simulink model "simulation"  (R2023a)
settings: Solver=ode4  StartTime=0.0  StopTime=simulation_time_end  FixedStep=simulation_time_step  RelTol=1e-3
values from neighbouring files (symbols this model uses):
  b = 0.0043    [code_Q2.m]
  J = 0.005    [code_Q2.m]
  K_b = 0.024    [code_Q2.m]
  K_m = 24e-3    (= 0.024)    [code_Q2.m]
  K_p = my_K_p    [code_Q2.m]
  K_u = 1.2    [code_Q2.m]
  L_a = 0.26e-3    (= 0.00026)    [code_Q2.m]
  N_r = 4.9    [code_Q2.m]
  R_a = 2.2    [code_Q2.m]
  simulation_time_start = 1    [code_Q2.m]
  T_d = 0    [code_Q2.m]
  theta_ref = pi/4    (= 0.785398163397)    [code_Q2.m]
settings Model: Creator=אלמוג  LastModifiedBy=אלמוג

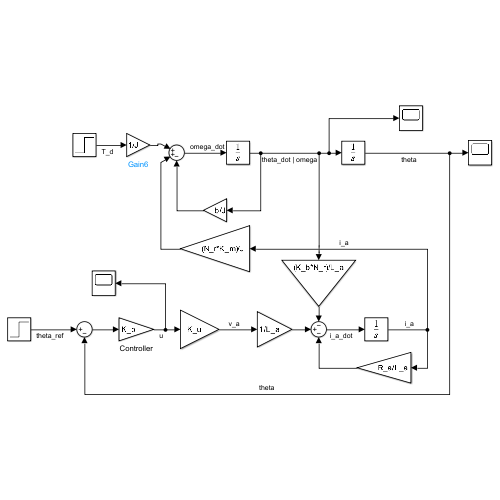
[thumbnail: Simulink's stored preview of the top-level diagram]
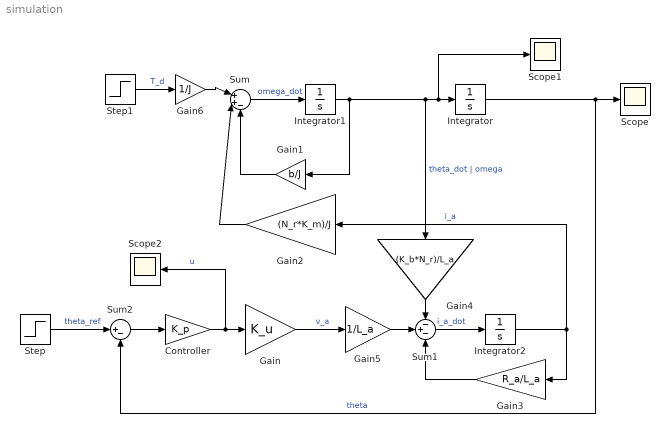
== system simulation ==
  Controller : Gain  Gain=K_p
  Gain : Gain  Gain=K_u
  Gain1 : Gain  Gain=b/J
  Gain2 : Gain  Gain=(N_r*K_m)/J
  Gain3 : Gain  Gain=R_a/L_a
  Gain4 : Gain  Gain=(K_b*N_r)/L_a
  Gain5 : Gain  Gain=1/L_a
  Gain6 : Gain  Gain=1/J
  Integrator : Integrator
  Integrator1 : Integrator
  Integrator2 : Integrator
  Scope : Scope
  Scope1 : Scope
  Scope2 : Scope
  Step : Step  Time=simulation_time_start  After=theta_ref  SampleTime=0
  Step1 : Step  Time=simulation_time_start  After=T_d  SampleTime=0
  Sum : Sum  Inputs=|++-
  Sum1 : Sum  Inputs=-+-
  Sum2 : Sum  Inputs=|+-
  wires:
  Controller/1 -> Gain/1, Scope2/1  "u"
  Gain/1 -> Gain5/1  "v_a"
  Integrator/1 -> Sum2/2, Scope/1  "theta"
  Integrator1/1 -> Integrator/1, Scope1/1, Gain4/1, Gain1/1  "theta_dot | omega"
  Sum/1 -> Integrator1/1  "omega_dot"
  Gain1/1 -> Sum/3
  Gain2/1 -> Sum/2
  Integrator2/1 -> Gain2/1, Gain3/1  "i_a"
  Sum1/1 -> Integrator2/1  "i_a_dot"
  Gain3/1 -> Sum1/3
  Gain4/1 -> Sum1/1
  Gain5/1 -> Sum1/2
  Step1/1 -> Gain6/1  "T_d"
  Gain6/1 -> Sum/1
  Sum2/1 -> Controller/1
  Step/1 -> Sum2/1  "theta_ref"
